simulink model "LQR_sim_discrete"  (R2020b)
settings: Solver=ode45  StartTime=0.0  StopTime=10  FixedStep=0.00001  RelTol=1e-3  EnableMultiTasking=on
values from neighbouring files (symbols this model uses):
  h = 0.01    [LQR_discrete.m]    (also in system_test.m = 0.001)
  Kd = place(sysd.A, sysd.B, poles_d)    [LQR_discrete.m]
  Ld = place(sysd.A',sysd.C',obs_poles_d).'    [LQR_discrete.m]
  sysd = c2d(sysc, h)    [linModelDT.m]
  Theta1_0 = 0    [LQR.m]    (also in LQR_discrete.m; simulation.m = 3.14159265359)
  Theta2_0 = 0.048    [LQR.m]    (also in LQR_discrete.m = 0.035; simulation.m = -1.57079632679)
  Thetad1_0 = 0    [LQR.m]    (also in LQR_discrete.m; simulation.m)
  Thetad2_0 = 0    [LQR.m]    (also in LQR_discrete.m; simulation.m)
settings Model: Creator=rbabuska  LastModifiedBy=fballast
settings DataIOCC: LimitDataPoints=on  SaveFormat=Array  ReturnWorkspaceOutputs=off  SignalLoggingName=sigsOut
settings OptimizationCC: BooleanDataType=off  ExpressionDepthLimit=2147483647  InitFltsAndDblsToZero=on  LifeSpan=inf
settings DebuggingCC: SaveWithParameterizedLinksMsg=none  SignalResolutionControl=TryResolveAllWithWarning  MultiTaskDSMMsg=warning  MultiTaskCondExecSysMsg=none  AllowSymbolicDim=off  StateNameClashWarn=warning  SFUnexpectedBacktrackingDiag=warning  SFNoUnconditionalDefaultTransitionDiag=warning  SFExecutionAtInitializationDiag=none  ArithmeticOperatorsInVariantConditions=warning
settings HardwareCC: ProdBitPerPointer=32  ProdBitPerSizeT=32  ProdBitPerPtrDiffT=32  ProdLargestAtomicFloat=None  ProdIntDivRoundTo=Undefined  ProdEndianess=Unspecified  ProdWordSize=32  ProdHWDeviceType=32-bit Generic  TargetUnknown=on
settings ModelReferenceCC: PropagateSignalLabelsOutOfModel=off
settings SFSimCC: SimUseLocalCustomCode=off  CustomCodeUndefinedFunction=UseInterfaceOnly
settings RTWCC: RTWUseLocalCustomCode=off
settings CodeAppCC: StateflowObjectComments=on
settings GRTTargetCC: TargetFcnLib=ansi_tfl_tmw.mat  TargetLangStandard=C89/C90 (ANSI)  CombineOutputUpdateFcns=off  GRTInterface=on
settings ConfigComp: CovMetricSettings=dw  CovSaveCumulativeToWorkspaceVar=on  CovSaveSingleToWorkspaceVar=on  CovExternalEMLEnable=off

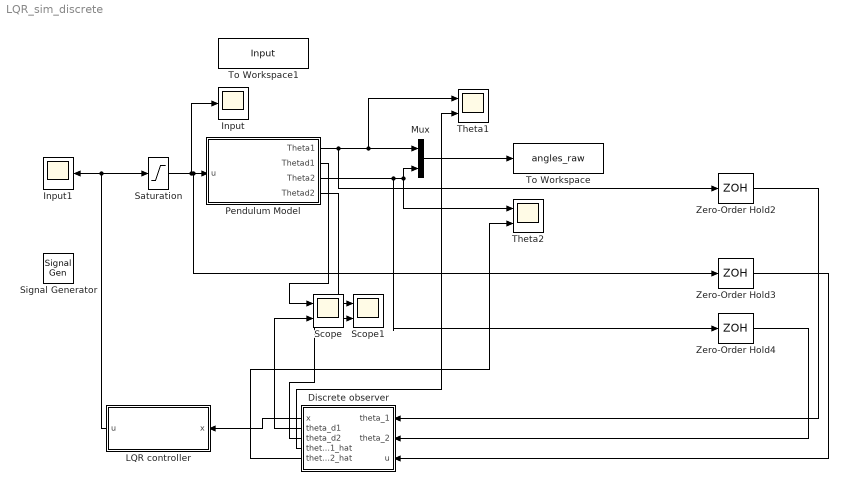
== system LQR_sim_discrete ==
  Discrete observer : Subsystem
  Input : Scope
  Input1 : Scope
  LQR controller : Subsystem
  Mux : Mux  Inputs=2
  Pendulum Model : Subsystem
  Saturation : Saturate  UpperLimit=1  LowerLimit=-1
  Scope : Scope  NumInputPorts=2
  Scope1 : Scope  NumInputPorts=2
  Signal Generator : SignalGenerator  Amplitude=0.7  Frequency=3  Units=rad/sec
  Theta1 : Scope  NumInputPorts=2
  Theta2 : Scope  NumInputPorts=2
  To Workspace : ToWorkspace  VariableName=angles_raw  SaveFormat=Timeseries  SampleTime=-1
  To Workspace1 : ToWorkspace  VariableName=Input  SaveFormat=Timeseries  SampleTime=-1
  Zero-Order Hold2 : ZeroOrderHold  SampleTime=h
  Zero-Order Hold3 : ZeroOrderHold  SampleTime=h
  Zero-Order Hold4 : ZeroOrderHold  SampleTime=h
  wires:
  Mux/1 -> To Workspace/1
  LQR controller/1(u) -> Saturation/1, Input1/1
  Pendulum Model/2(Thetad1) -> Scope/1
  Discrete observer/2(theta_d1) -> Scope/2
  Discrete observer/3(theta_d2) -> Scope1/2
  Pendulum Model/4(Thetad2) -> Scope1/1
  Discrete observer/4(theta_1_hat) -> Theta1/2
  Discrete observer/5(theta_2_hat) -> Theta2/2
  Discrete observer/1(x) -> LQR controller/1(x)
  Pendulum Model/1(Theta1) -> Zero-Order Hold2/1, Mux/1, Theta1/1
  Pendulum Model/3(Theta2) -> Zero-Order Hold4/1, Mux/2, Theta2/1
  Saturation/1 -> Input/1, Zero-Order Hold3/1, Pendulum Model/1(u)
  Zero-Order Hold2/1 -> Discrete observer/1(theta_1)
  Zero-Order Hold3/1 -> Discrete observer/3(u)
  Zero-Order Hold4/1 -> Discrete observer/2(theta_2)

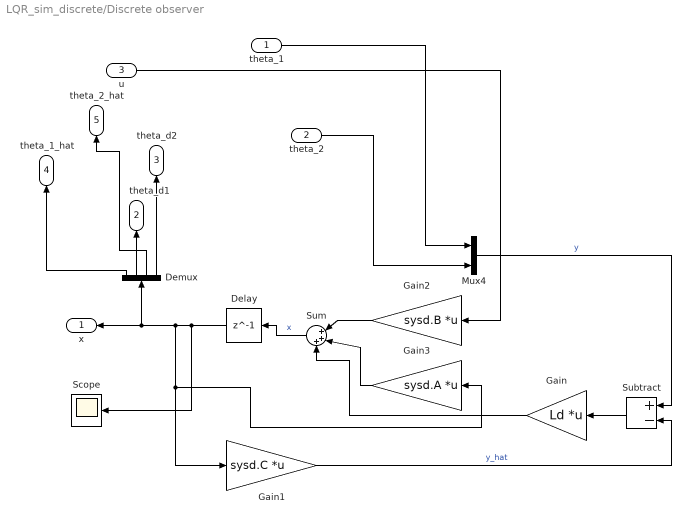
== system LQR_sim_discrete/Discrete observer ==
  theta_1 : Inport
  theta_2 : Inport  Port=2
  u : Inport  Port=3
  Delay : Delay  DelayLength=1
  Demux : Demux
  Gain : Gain  Gain=Ld  Multiplication=Matrix(K*u) (u vector)
  Gain1 : Gain  Gain=sysd.C  Multiplication=Matrix(K*u) (u vector)
  Gain2 : Gain  Gain=sysd.B  Multiplication=Matrix(K*u) (u vector)
  Gain3 : Gain  Gain=sysd.A  Multiplication=Matrix(K*u) (u vector)
  Mux4 : Mux  Inputs=2
  Scope : Scope
  Subtract : Sum  Inputs=+-
  Sum : Sum  Inputs=|+++
  x : Outport
  theta_d1 : Outport  Port=2
  theta_d2 : Outport  Port=3
  theta_1_hat : Outport  Port=4
  theta_2_hat : Outport  Port=5
  wires:
  Gain1/1 -> Subtract/2  "y_hat"
  theta_2/1 -> Mux4/2
  Subtract/1 -> Gain/1
  Gain/1 -> Sum/3
  Gain2/1 -> Sum/1
  Sum/1 -> Delay/1  "x"
  Mux4/1 -> Subtract/1  "y"
  Gain3/1 -> Sum/2
  u/1 -> Gain2/1
  theta_1/1 -> Mux4/1
  Demux/2 -> theta_d1/1
  Demux/4 -> theta_d2/1
  Demux/1 -> theta_1_hat/1
  Demux/3 -> theta_2_hat/1
  Delay/1 -> Scope/1, Demux/1, x/1, Gain3/1, Gain1/1

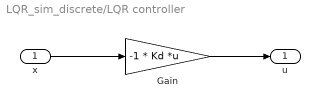
== system LQR_sim_discrete/LQR controller ==
  x : Inport
  Gain : Gain  Gain=-1 * Kd  Multiplication=Matrix(K*u) (u vector)
  u : Outport
  wires:
  x/1 -> Gain/1
  Gain/1 -> u/1

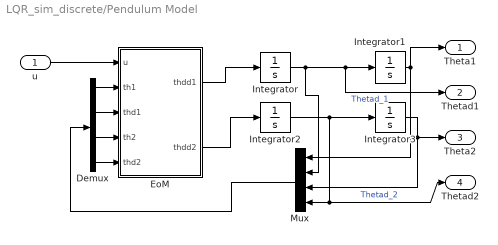
== system LQR_sim_discrete/Pendulum Model ==
  u : Inport
  Demux : Demux
  EoM : MATLAB Function  TreatAsAtomicUnit=on
  Integrator : Integrator  InitialCondition=Thetad1_0  ContinuousStateAttributes='Theta1'
  Integrator1 : Integrator  InitialCondition=Theta1_0  ContinuousStateAttributes='Theta1'
  Integrator2 : Integrator  InitialCondition=Thetad2_0  ContinuousStateAttributes='Theta1'
  Integrator3 : Integrator  InitialCondition=Theta2_0  ContinuousStateAttributes='Theta1'
  Mux : Mux
  Theta1 : Outport
  Thetad1 : Outport  Port=2
  Theta2 : Outport  Port=3
  Thetad2 : Outport  Port=4
  wires:
  Integrator1/1 -> Mux/1, Theta1/1
  Integrator/1 -> Mux/2, Integrator1/1, Thetad1/1  "Thetad_1"
  EoM/2(thdd2) -> Integrator2/1
  Integrator2/1 -> Thetad2/1, Mux/4, Integrator3/1  "Thetad_2"
  Integrator3/1 -> Theta2/1, Mux/3
  u/1 -> EoM/1(u)
  EoM/1(thdd1) -> Integrator/1
  Demux/1 -> EoM/2(th1)
  Demux/2 -> EoM/3(thd1)
  Demux/3 -> EoM/4(th2)
  Demux/4 -> EoM/5(thd2)
  Mux/1 -> Demux/1

== matlab function LQR_sim_discrete/Pendulum Model/EoM ==
  data: u input; thdd1 output; th1 input; thd1 input; th2 input; thd2 input; model_par parameter; thdd2 output
function [thdd1, thdd2] = fcn(u, th1, thd1, th2, thd2, model_par)
thdd1 = -model_par.a11*thd1 - model_par.a12 * u;
F = -model_par.c2*model_par.l1*model_par.m2*sin(thd2)*thd1^2 - model_par.b2*thd2 + model_par.c2*model_par.g*model_par.m2*sin(th1 + th2);
M21 = model_par.m2*model_par.c2^2 + model_par.l1*model_par.m2*cos(thd2)*model_par.c2 + model_par.J2;
M22 = model_par.m2*model_par.c2^2 + model_par.J2;
thdd2 = F/M22 - M21/M22 * thdd1;
